simulink model "testes_com_trajetorias"  (R2016a)
settings: Solver=ode14x  StartTime=0.0  StopTime=30  FixedStep=0.001  RelTol=1e-3
InitFcn:
  | clear all;
  | Kpx = 10;
  | Kix = 25;
  | Kpy = 10;
  | Kiy = 25;
  | Kvphi = 3;
  | Kpphi = 2.25;
  | 
  | Kem = 0.0059;
  | Kti = 0.0059;
  | Vd = 5.4;
  | R = 1.71;
  | r = 0.072;
  | eta = 0.83;
  | N = 19;
  | 
  | Jw = 8.1e-4;
  | 
  | mi = 0.25;
  | b = .1;
  | 
  | Ts = 0.01;
  | 
  | 
  | alpha1 = 0;
  | alpha2 = 120*pi/180;
  | alpha3 = 240*pi/180;
  | g = 9.8;
  | vs = 6e-10;
  | M = 1.83;
  | l1 = 0.09;
  | l2 = 0.09;
  | l3 = 0.09;
  | r1 = 0.072;
  | r2 = 0.072;
  | r3 = 0.072;
  | kt = 0.0059;
  | kem = 0.0059;
  | N = 19;
  | L = 0.00011;
  | R = 1.71;
  | Jm1 = 3.88e-7;
  | Jm2 = 3.88e-7;
  | Jm3 = 3.88e-7;
  | J1 = 8.1e-4;
  | J2 = 8.1e-4;
  | J3 = 8.1e-4;
  | J = 2.125;
  | eta = 0.83;
  | freq = 1000; % varia entre 2.5kHz e 5Mhz
  | mic = 0.25;
  | mis = 0.25;
  | sigma0 = 100;
  | sigma1 = 0.1;
  | sigma2 = 0.1;
  | 
  | mi = 0.25;
  | b = .1;
  | 
  | kctr = kt*5.4*eta*N/(R*r1)
libraries: simulink x2
settings Model: Creator=Pichau  LastModifiedBy=Pichau

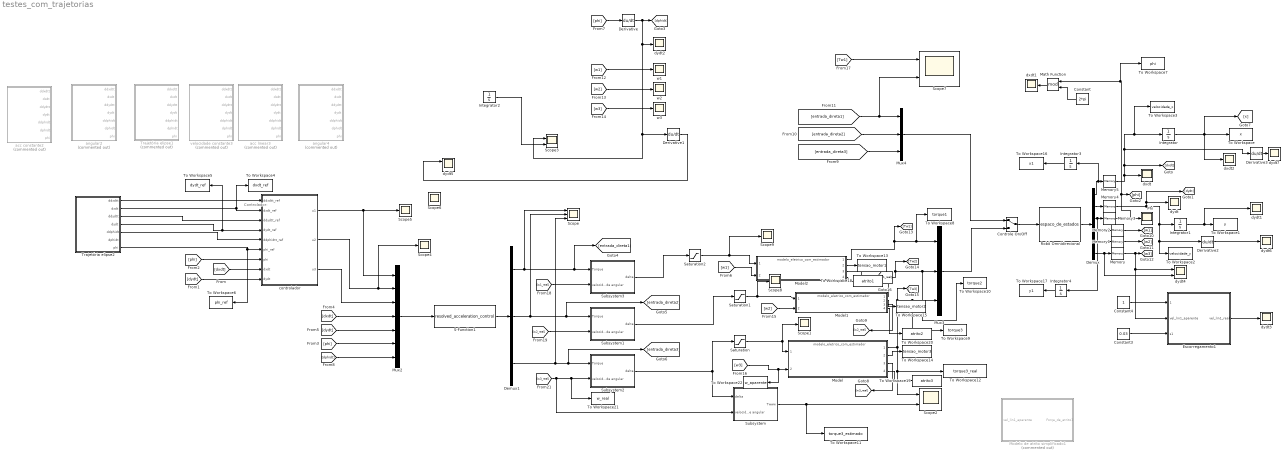
== system testes_com_trajetorias ==
  note: Controlador:
  Constant : Constant  Value=2*pi
  Constant3 : Constant  Value=0.03
  Constant4 : Constant
  Controle On/Off : ManualSwitch
  Demux : Demux  Outputs=6
  Demux1 : Demux  Outputs=3
  Derivative{,1..3} (4 alike) : Derivative
  Escorregamento1 : Subsystem
  Integrator : Integrator  InitialCondition=0.3
  Integrator{1..4} (4 alike) : Integrator
  Math Function : Math  Operator=mod  SaturateOnIntegerOverflow=on
  Memory{,1..2,4..5} (5 alike) : Memory
  Memory3 : Memory  X0=pi/2
  Model : ModelReference  ModelNameDialog=modelo_eletrico_com_estimador  SimulationMode=Normal  ModelReferenceVersion=1.40
  Model1 : ModelReference  ModelNameDialog=modelo_eletrico_com_estimador  SimulationMode=Normal  ModelReferenceVersion=1.40
  Model2 : ModelReference  ModelNameDialog=modelo_eletrico_com_estimador  SimulationMode=Normal  ModelReferenceVersion=1.40
  Modelo de atrito simplificado1 : Subsystem  Commented=on
  Mux2 : Mux  Inputs=7
  Mux3 : Mux  Inputs=3
  Mux4 : Mux  Inputs=3
  Phi : Scope
  Robô Omnidirecional : S-Function  FunctionName=espaco_de_estados  Parameters=r,m,Jw,J,L  SFunctionDeploymentMode=off  EnableBusSupport=off  mask{r=0.072, m=1.71, Jw=8.1e-4, J=2.125, L=0.09}
      mask prompts: r "r (m)"; m "m (Kg)"; Jw "Jw (Kg*m^2)"; J "J (Kg*m^2)"; L "L (m)"
      mask Display: image(imread('Robot_omnidirectional_drive.png'));
  S-Function1 : S-Function  FunctionName=resolved_acceleration_control  Parameters=r,L,m,J,Jw  SFunctionDeploymentMode=off  EnableBusSupport=off  mask{r=0.072, L=0.09, m=1.71, J=2.125, Jw=8.1e-4}
  Saturation : Saturate  UpperLimit=1  LowerLimit=-1
  Saturation1 : Saturate  UpperLimit=1  LowerLimit=-1
  Saturation2 : Saturate  UpperLimit=1  LowerLimit=-1
  Scope : Scope  NumInputPorts=3
  Scope{1,4..6,8..9} (6 alike) : Scope
  Scope2 : Scope  NumInputPorts=2
  Scope3 : Scope  NumInputPorts=2
  Scope7 : Scope  NumInputPorts=2
  Subsystem : Subsystem
  Subsystem1 : Subsystem
  Subsystem2 : Subsystem
  Subsystem3 : Subsystem
  To Workspace : ToWorkspace  VariableName=x  SaveFormat=Timeseries  SampleTime=-1
  To Workspace1 : ToWorkspace  VariableName=y  SaveFormat=Timeseries  SampleTime=-1
  To Workspace10 : ToWorkspace  VariableName=torque2  SaveFormat=Timeseries  SampleTime=-1
  To Workspace11 : ToWorkspace  VariableName=torque3_estimado  SaveFormat=Timeseries  SampleTime=-1
  To Workspace12 : ToWorkspace  VariableName=torque3_real  SaveFormat=Timeseries  SampleTime=-1
  To Workspace13 : ToWorkspace  VariableName=tensao_motor1  SaveFormat=Timeseries  SampleTime=-1
  To Workspace14 : ToWorkspace  VariableName=tensao_motor3  SaveFormat=Timeseries  SampleTime=-1
  To Workspace15 : ToWorkspace  VariableName=tensao_motor2  SaveFormat=Timeseries  SampleTime=-1
  To Workspace16 : ToWorkspace  VariableName=x1  SaveFormat=Timeseries  SampleTime=-1
  To Workspace17 : ToWorkspace  VariableName=y1  SaveFormat=Timeseries  SampleTime=-1
  To Workspace18 : ToWorkspace  VariableName=atrito1  SaveFormat=Timeseries  SampleTime=-1
  To Workspace19 : ToWorkspace  VariableName=atrito3  SaveFormat=Timeseries  SampleTime=-1
  To Workspace2 : ToWorkspace  VariableName=velocidade_y  SaveFormat=Timeseries  SampleTime=-1
  To Workspace20 : ToWorkspace  VariableName=atrito2  SaveFormat=Timeseries  SampleTime=-1
  To Workspace21 : ToWorkspace  VariableName=w_real  SaveFormat=Timeseries  SampleTime=-1
  To Workspace22 : ToWorkspace  VariableName=w_aparente  SaveFormat=Timeseries  SampleTime=-1
  To Workspace3 : ToWorkspace  VariableName=velocidade_x  SaveFormat=Timeseries  SampleTime=-1
  To Workspace4 : ToWorkspace  VariableName=dxdt_ref  SaveFormat=Timeseries  SampleTime=-1
  To Workspace5 : ToWorkspace  VariableName=dydt_ref  SaveFormat=Timeseries  SampleTime=-1
  To Workspace6 : ToWorkspace  VariableName=phi_ref  SaveFormat=Timeseries  SampleTime=-1
  To Workspace7 : ToWorkspace  VariableName=phi  SaveFormat=Timeseries  SampleTime=-1
  To Workspace8 : ToWorkspace  VariableName=torque1  SaveFormat=Timeseries  SampleTime=-1
  To Workspace9 : ToWorkspace  VariableName=torque3  SaveFormat=Timeseries  SampleTime=-1
  Trajetória elipse1 : Subsystem  Commented=on
  Trajetória elipse2 : Subsystem
  acc constante2 : Subsystem  Commented=on
  acc linear3 : Subsystem  Commented=on
  angular2 : Subsystem  Commented=on
  angular4 : Subsystem  Commented=on
  controlador : Subsystem
  dxdt : Scope
  dxdt1 : Scope
  dxdt2 : Scope
  dydt{,1..3,6..7} (6 alike) : Scope
  dydt4 : Scope  NumInputPorts=2
  dydt5 : Scope  NumInputPorts=2
  velocidade constante3 : Subsystem  Commented=on
  w1 : Scope
  w2 : Scope
  w3 : Scope
  wires:
  Robô Omnidirecional/1 -> Demux/1
  Integrator1/1 -> dydt1/1, To Workspace1/1
  Integrator/1 -> dxdt2/1, [x], To Workspace/1
  Trajetória elipse2/2(dxdt) -> controlador/2(dxdt_ref), To Workspace4/1
  Trajetória elipse2/1(ddxdtt) -> controlador/1(ddxdtt_ref)
  Trajetória elipse2/4(dydt) -> To Workspace5/1, controlador/4(dydt_ref)
  Trajetória elipse2/3(ddydtt) -> controlador/3(ddydtt_ref)
  Trajetória elipse2/7(phi) -> To Workspace6/1, controlador/6(phi_ref)
  Trajetória elipse2/5(ddphidt) -> controlador/5(ddphidtt_ref)
  [dxdt] -> controlador/8(dxdt)
  [dydt] -> controlador/9(dydt)
  [phi] -> controlador/7(phi)
  Mux2/1 -> S-Function1/1
  Derivative/1 -> Scope3/1, Derivative1/1, dydt2/1, [dphidt]
  S-Function1/1 -> Demux1/1
  Mux3/1 -> Controle On/Off/2
  Controle On/Off/1 -> Robô Omnidirecional/1
  [w3] -> w3/1
  [w2] -> w2/1
  [w1] -> w1/1
  Demux/1 -> Integrator3/1, Memory5/1
  Demux/2 -> Memory4/1
  [phi] -> Derivative/1
  [dxdt] -> Mux2/4
  [dydt] -> Mux2/5
  [phi] -> Mux2/6
  [dphidt] -> Mux2/7
  Demux/4 -> Memory2/1
  Demux/5 -> Memory1/1
  Demux/6 -> dydt4/2, Memory/1
  Model/1 -> [Tw3], Mux3/3, To Workspace9/1, Scope2/1, To Workspace12/1
  Model1/1 -> [Tw2], To Workspace10/1, Mux3/2
  Model2/1 -> [Tw1], To Workspace8/1, Mux3/1
  Mux4/1 -> Controle On/Off/1
  Demux1/1 -> Scope/1, Subsystem3/1(Torque), [entrada_direta1]
  Subsystem1/1(delta) -> Saturation1/1
  Subsystem3/1(delta) -> Saturation2/1
  [w1_real] -> Subsystem3/2(velocidade angular)
  [w2_real] -> Subsystem1/2(velocidade angular)
  [w3_real] -> Subsystem/2(velocidade angular), To Workspace21/1, Subsystem2/2(velocidade angular)
  Constant3/1 -> Escorregamento1/3(s1)
  Constant4/1 -> Escorregamento1/1(1)
  Escorregamento1/1("vel_lin1_real ") -> dydt3/1
  Memory/1 -> Escorregamento1/2("vel_lin1_aparente "), dydt4/1, [w3]
  Memory1/1 -> [w2]
  Memory2/1 -> [w1]
  Memory4/1 -> To Workspace2/1, Derivative2/1, Integrator1/1, [dydt], dydt/1
  Memory5/1 -> [dxdt], Derivative3/1, To Workspace3/1, Integrator/1, dxdt/1
  Subsystem2/1(delta) -> Subsystem/1(delta), Saturation/1
  Subsystem/1(Twww) -> To Workspace11/1, Scope2/2
  Demux1/2 -> Scope/2, Subsystem1/1(Torque), [entrada_direta2]
  Demux1/3 -> Scope/3, [entrada_direta3], Subsystem2/1(Torque)
  Math Function/1 -> dxdt1/1
  Constant/1 -> Math Function/2
  Memory3/1 -> Phi/1, [phi], To Workspace7/1, Math Function/1
  Saturation/1 -> Scope1/1, Model/1
  Saturation1/1 -> Scope8/1, Model1/1
  [entrada_direta3] -> Mux4/3
  [entrada_direta2] -> Mux4/2
  Integrator2/1 -> Scope3/2
  Derivative1/1 -> dydt5/1
  Derivative2/1 -> dydt6/1
  Derivative3/1 -> dydt7/1
  controlador/2(u2) -> Scope4/1, Mux2/2
  controlador/1(u1) -> Mux2/1, Scope5/1
  controlador/3(u3) -> Mux2/3
  [w1] -> Model2/2
  [w2] -> Model1/2
  [w3] -> To Workspace22/1, Model/2
  [Tw1] -> Scope7/1
  [entrada_direta1] -> Scope7/2, Mux4/1
  Saturation2/1 -> Scope9/1, Model2/1
  Model2/2 -> To Workspace13/1
  Model1/2 -> To Workspace15/1
  Model/2 -> To Workspace14/1
  Integrator3/1 -> To Workspace16/1
  Demux/3 -> Integrator4/1, Memory3/1
  Integrator4/1 -> To Workspace17/1
  Model/3 -> [w3_real]
  Model1/3 -> [w2_real]
  Model2/3 -> [w1_real]
  Model2/4 -> To Workspace18/1
  Model1/4 -> To Workspace20/1
  Model/4 -> To Workspace19/1

== system testes_com_trajetorias/Escorregamento1 ==
  1 : Inport
  "vel_lin1_aparente " : Inport  Port=2
  s1 : Inport  Port=3
  Fcn : Fcn  Expr=1/u[1]
  Product : Product  RndMeth=Zero
  Sum3 : Sum  Inputs=+|+
  Sum4 : Sum  Inputs=|+-
  Switch : Switch
  "vel_lin1_real " : Outport
  wires:
  s1/1 -> Switch/2, Sum3/1, Sum4/2
  1/1 -> Sum3/2, Sum4/1
  Sum4/1 -> Fcn/1
  Fcn/1 -> Switch/1
  Sum3/1 -> Switch/3
  Switch/1 -> Product/2
  "vel_lin1_aparente "/1 -> Product/1
  Product/1 -> "vel_lin1_real "/1

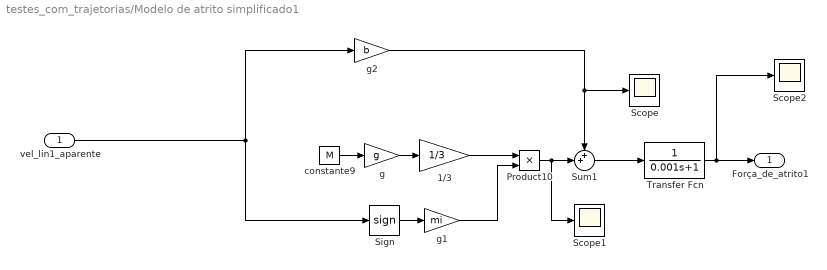
== system testes_com_trajetorias/Modelo de atrito simplificado1 ==
  vel_lin1_aparente : Inport
  1/3 : Gain  Gain=1/3
  Product10 : Product  RndMeth=Zero
  Scope : Scope
  Scope1 : Scope
  Scope2 : Scope
  Sign : Signum
  Sum1 : Sum  Inputs=++|
  Transfer Fcn : TransferFcn  Denominator=[0.001 1]
  constante9 : Constant  Value=M
  g : Gain  Gain=g
  g1 : Gain  Gain=mi
  g2 : Gain  Gain=b
  Força_de_atrito1 : Outport
  wires:
  Transfer Fcn/1 -> Força_de_atrito1/1, Scope2/1
  g2/1 -> Scope/1, Sum1/1
  Sum1/1 -> Transfer Fcn/1
  Sign/1 -> g1/1
  vel_lin1_aparente/1 -> Sign/1, g2/1
  Product10/1 -> Sum1/2, Scope1/1
  g1/1 -> Product10/2
  1/3/1 -> Product10/1
  g/1 -> 1/3/1
  constante9/1 -> g/1

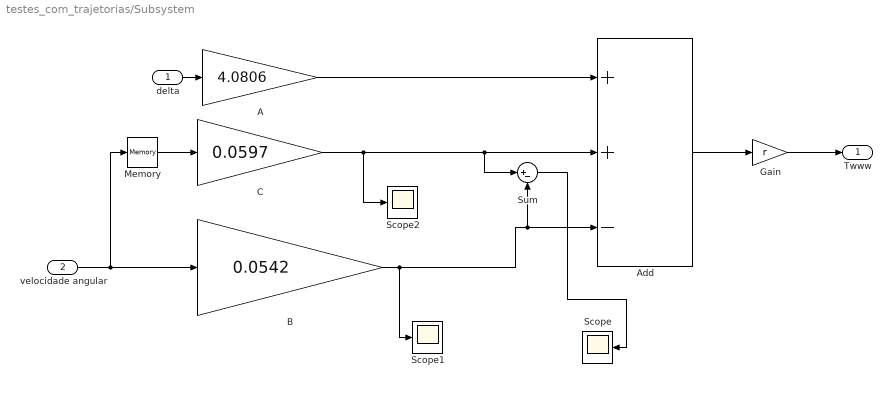
== system testes_com_trajetorias/Subsystem ==
  delta : Inport
  velocidade angular : Inport  Port=2
  A : Gain  Gain=4.0806
  Add : Sum  Inputs=++-
  B : Gain  Gain=0.0542
  C : Gain  Gain=0.0597
  Gain : Gain  Gain=r
  Memory : Memory
  Scope : Scope
  Scope1 : Scope
  Scope2 : Scope
  Sum : Sum  Inputs=|+-
  Twww : Outport
  wires:
  Add/1 -> Gain/1
  delta/1 -> A/1
  velocidade angular/1 -> Memory/1, B/1
  A/1 -> Add/1
  Memory/1 -> C/1
  Gain/1 -> Twww/1
  C/1 -> Scope2/1, Sum/1, Add/2
  Sum/1 -> Scope/1
  B/1 -> Scope1/1, Add/3, Sum/2

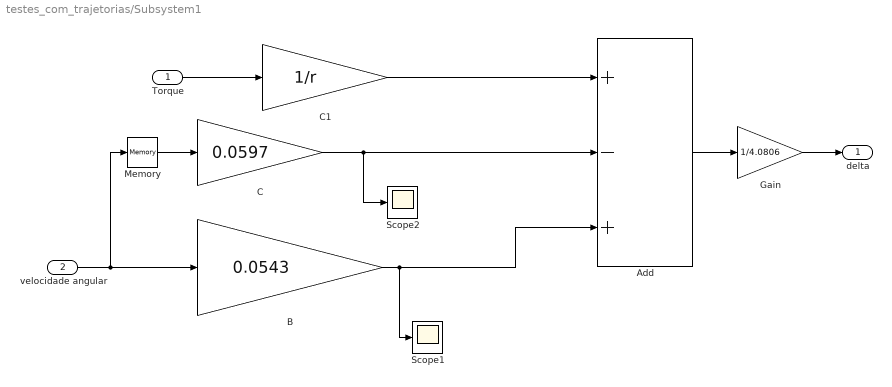
== system testes_com_trajetorias/Subsystem1 ==
  Torque : Inport
  velocidade angular : Inport  Port=2
  Add : Sum  Inputs=+-+
  B : Gain  Gain=0.0543
  C : Gain  Gain=0.0597
  C1 : Gain  Gain=1/r
  Gain : Gain  Gain=1/4.0806
  Memory : Memory
  Scope1 : Scope
  Scope2 : Scope
  delta : Outport
  wires:
  C1/1 -> Add/1
  Add/1 -> Gain/1
  velocidade angular/1 -> Memory/1, B/1
  Torque/1 -> C1/1
  Memory/1 -> C/1
  Gain/1 -> delta/1
  C/1 -> Scope2/1, Add/2
  B/1 -> Scope1/1, Add/3

== system testes_com_trajetorias/Subsystem2 ==
  Torque : Inport
  velocidade angular : Inport  Port=2
  Add : Sum  Inputs=+-+
  B : Gain  Gain=0.0543
  C : Gain  Gain=0.0597
  C1 : Gain  Gain=1/r
  Gain : Gain  Gain=1/4.0806
  Memory : Memory
  Scope1 : Scope
  Scope2 : Scope
  delta : Outport
  wires:
  B/1 -> Add/3, Scope1/1
  C/1 -> Add/2, Scope2/1
  Gain/1 -> delta/1
  Memory/1 -> C/1
  Torque/1 -> C1/1
  velocidade angular/1 -> B/1, Memory/1
  Add/1 -> Gain/1
  C1/1 -> Add/1

== system testes_com_trajetorias/Subsystem3 ==
  Torque : Inport
  velocidade angular : Inport  Port=2
  Add : Sum  Inputs=+-+
  B : Gain  Gain=0.0543
  C : Gain  Gain=0.0597
  C1 : Gain  Gain=1/r
  Gain : Gain  Gain=1/4.0806
  Memory : Memory
  Scope1 : Scope
  Scope2 : Scope
  delta : Outport
  wires:
  B/1 -> Add/3, Scope1/1
  C/1 -> Add/2, Scope2/1
  Gain/1 -> delta/1
  Memory/1 -> C/1
  Torque/1 -> C1/1
  velocidade angular/1 -> B/1, Memory/1
  Add/1 -> Gain/1
  C1/1 -> Add/1

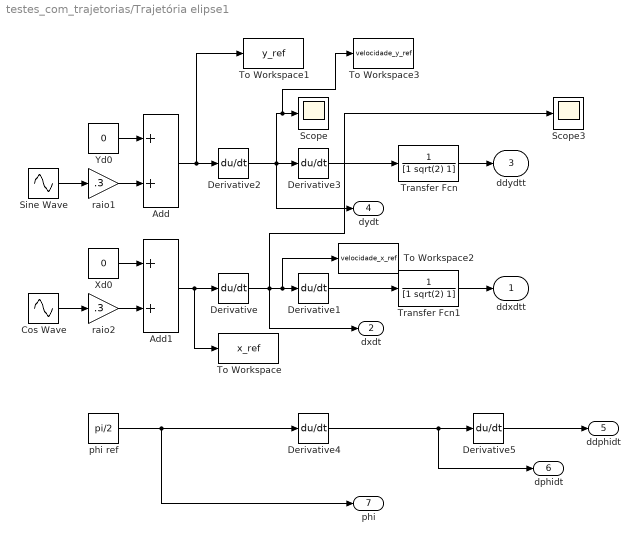
== system testes_com_trajetorias/Trajetória elipse1 ==
  Add : Sum
  Add1 : Sum
  Cos Wave : Sin  Frequency=0.3  Phase=pi/2  SampleTime=0
  Derivative{,1..5} (6 alike) : Derivative
  Scope : Scope
  Scope3 : Scope
  Sine Wave : Sin  Frequency=0.3  SampleTime=0
  To Workspace : ToWorkspace  VariableName=x_ref  SaveFormat=Timeseries  SampleTime=-1
  To Workspace1 : ToWorkspace  VariableName=y_ref  SaveFormat=Timeseries  SampleTime=-1
  To Workspace2 : ToWorkspace  VariableName=velocidade_x_ref  SaveFormat=Timeseries  SampleTime=-1
  To Workspace3 : ToWorkspace  VariableName=velocidade_y_ref  SaveFormat=Timeseries  SampleTime=-1
  Transfer Fcn : TransferFcn  Denominator=[1 sqrt(2) 1]
  Transfer Fcn1 : TransferFcn  Denominator=[1 sqrt(2) 1]
  Xd0 : Constant  Value=0
  Yd0 : Constant  Value=0
  phi ref : Constant  Value=pi/2
  raio1 : Gain  Gain=.3
  raio2 : Gain  Gain=.3
  ddxdtt : Outport
  dxdt : Outport  Port=2
  ddydtt : Outport  Port=3
  dydt : Outport  Port=4
  ddphidt : Outport  Port=5
  dphidt : Outport  Port=6
  phi : Outport  Port=7
  wires:
  Derivative4/1 -> dphidt/1, Derivative5/1
  phi ref/1 -> phi/1, Derivative4/1
  Yd0/1 -> Add/1
  Xd0/1 -> Add1/1
  Cos Wave/1 -> raio2/1
  raio2/1 -> Add1/2
  Add1/1 -> Derivative/1, To Workspace/1
  Add/1 -> Derivative2/1, To Workspace1/1
  raio1/1 -> Add/2
  Sine Wave/1 -> raio1/1
  Derivative/1 -> dxdt/1, Derivative1/1, To Workspace2/1, Scope3/1
  Derivative2/1 -> dydt/1, Scope/1, To Workspace3/1, Derivative3/1
  Derivative3/1 -> Transfer Fcn/1
  Derivative1/1 -> Transfer Fcn1/1
  Derivative5/1 -> ddphidt/1
  Transfer Fcn/1 -> ddydtt/1
  Transfer Fcn1/1 -> ddxdtt/1

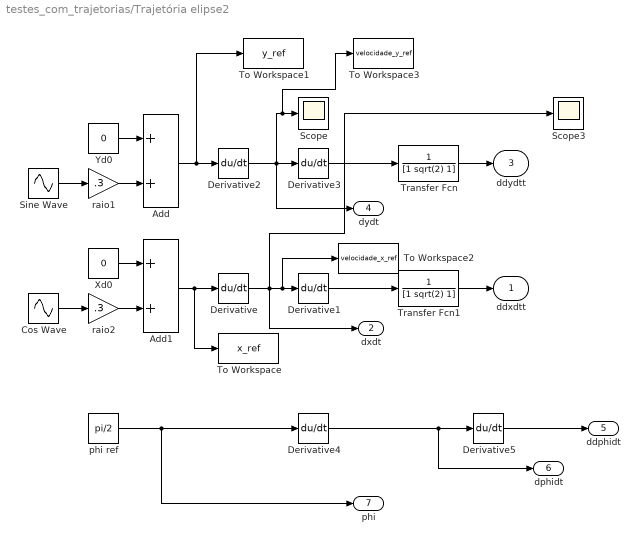
== system testes_com_trajetorias/Trajetória elipse2 ==
  Add : Sum
  Add1 : Sum
  Cos Wave : Sin  Frequency=0.3  Phase=pi/2  SampleTime=0
  Derivative{,1..5} (6 alike) : Derivative
  Scope : Scope
  Scope3 : Scope
  Sine Wave : Sin  Frequency=0.3  SampleTime=0
  To Workspace : ToWorkspace  VariableName=x_ref  SaveFormat=Timeseries  SampleTime=-1
  To Workspace1 : ToWorkspace  VariableName=y_ref  SaveFormat=Timeseries  SampleTime=-1
  To Workspace2 : ToWorkspace  VariableName=velocidade_x_ref  SaveFormat=Timeseries  SampleTime=-1
  To Workspace3 : ToWorkspace  VariableName=velocidade_y_ref  SaveFormat=Timeseries  SampleTime=-1
  Transfer Fcn : TransferFcn  Denominator=[1 sqrt(2) 1]
  Transfer Fcn1 : TransferFcn  Denominator=[1 sqrt(2) 1]
  Xd0 : Constant  Value=0
  Yd0 : Constant  Value=0
  phi ref : Constant  Value=pi/2
  raio1 : Gain  Gain=.3
  raio2 : Gain  Gain=.3
  ddxdtt : Outport
  dxdt : Outport  Port=2
  ddydtt : Outport  Port=3
  dydt : Outport  Port=4
  ddphidt : Outport  Port=5
  dphidt : Outport  Port=6
  phi : Outport  Port=7
  wires:
  Transfer Fcn1/1 -> ddxdtt/1
  Transfer Fcn/1 -> ddydtt/1
  Derivative5/1 -> ddphidt/1
  Derivative1/1 -> Transfer Fcn1/1
  Derivative3/1 -> Transfer Fcn/1
  Derivative2/1 -> Derivative3/1, To Workspace3/1, Scope/1, dydt/1
  Derivative/1 -> Scope3/1, To Workspace2/1, Derivative1/1, dxdt/1
  Sine Wave/1 -> raio1/1
  raio1/1 -> Add/2
  Add/1 -> To Workspace1/1, Derivative2/1
  Add1/1 -> To Workspace/1, Derivative/1
  raio2/1 -> Add1/2
  Cos Wave/1 -> raio2/1
  Xd0/1 -> Add1/1
  Yd0/1 -> Add/1
  phi ref/1 -> Derivative4/1, phi/1
  Derivative4/1 -> Derivative5/1, dphidt/1

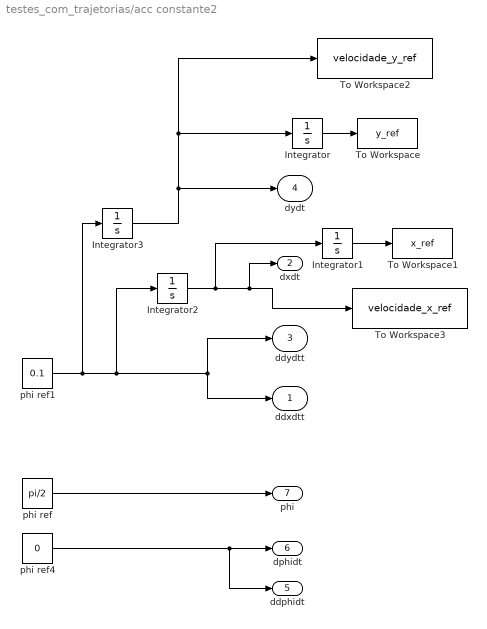
== system testes_com_trajetorias/acc constante2 ==
  Integrator{,1..3} (4 alike) : Integrator
  To Workspace : ToWorkspace  VariableName=y_ref  SaveFormat=Timeseries  SampleTime=-1
  To Workspace1 : ToWorkspace  VariableName=x_ref  SaveFormat=Timeseries  SampleTime=-1
  To Workspace2 : ToWorkspace  VariableName=velocidade_y_ref  SaveFormat=Timeseries  SampleTime=-1
  To Workspace3 : ToWorkspace  VariableName=velocidade_x_ref  SaveFormat=Timeseries  SampleTime=-1
  phi ref : Constant  Value=pi/2
  phi ref1 : Constant  Value=0.1
  phi ref4 : Constant  Value=0
  ddxdtt : Outport
  dxdt : Outport  Port=2
  ddydtt : Outport  Port=3
  dydt : Outport  Port=4
  ddphidt : Outport  Port=5
  dphidt : Outport  Port=6
  phi : Outport  Port=7
  wires:
  Integrator2/1 -> To Workspace3/1, dxdt/1, Integrator1/1
  Integrator1/1 -> To Workspace1/1
  Integrator/1 -> To Workspace/1
  Integrator3/1 -> dydt/1, To Workspace2/1, Integrator/1
  phi ref1/1 -> ddxdtt/1, ddydtt/1, Integrator2/1, Integrator3/1
  phi ref/1 -> phi/1
  phi ref4/1 -> ddphidt/1, dphidt/1

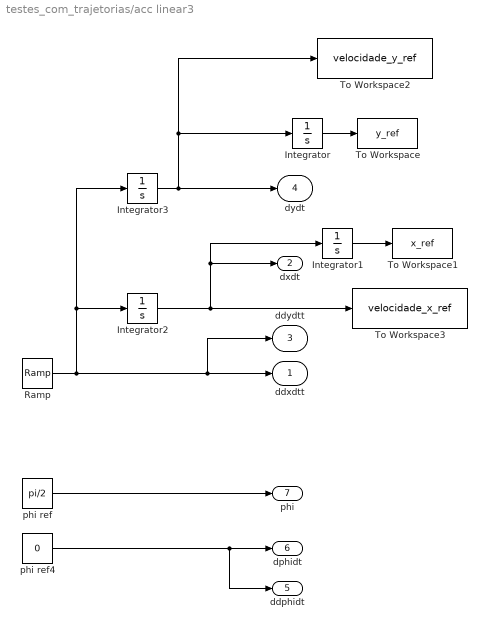
== system testes_com_trajetorias/acc linear3 ==
  Integrator{,1..3} (4 alike) : Integrator
  Ramp : simulink/Sources/Ramp  slope=0.01  start=0  X0=0
  To Workspace : ToWorkspace  VariableName=y_ref  SaveFormat=Timeseries  SampleTime=-1
  To Workspace1 : ToWorkspace  VariableName=x_ref  SaveFormat=Timeseries  SampleTime=-1
  To Workspace2 : ToWorkspace  VariableName=velocidade_y_ref  SaveFormat=Timeseries  SampleTime=-1
  To Workspace3 : ToWorkspace  VariableName=velocidade_x_ref  SaveFormat=Timeseries  SampleTime=-1
  phi ref : Constant  Value=pi/2
  phi ref4 : Constant  Value=0
  ddxdtt : Outport
  dxdt : Outport  Port=2
  ddydtt : Outport  Port=3
  dydt : Outport  Port=4
  ddphidt : Outport  Port=5
  dphidt : Outport  Port=6
  phi : Outport  Port=7
  wires:
  Integrator3/1 -> dydt/1, To Workspace2/1, Integrator/1
  Integrator1/1 -> To Workspace1/1
  Integrator/1 -> To Workspace/1
  Ramp/1 -> Integrator2/1, Integrator3/1, ddxdtt/1, ddydtt/1
  Integrator2/1 -> To Workspace3/1, dxdt/1, Integrator1/1
  phi ref/1 -> phi/1
  phi ref4/1 -> ddphidt/1, dphidt/1

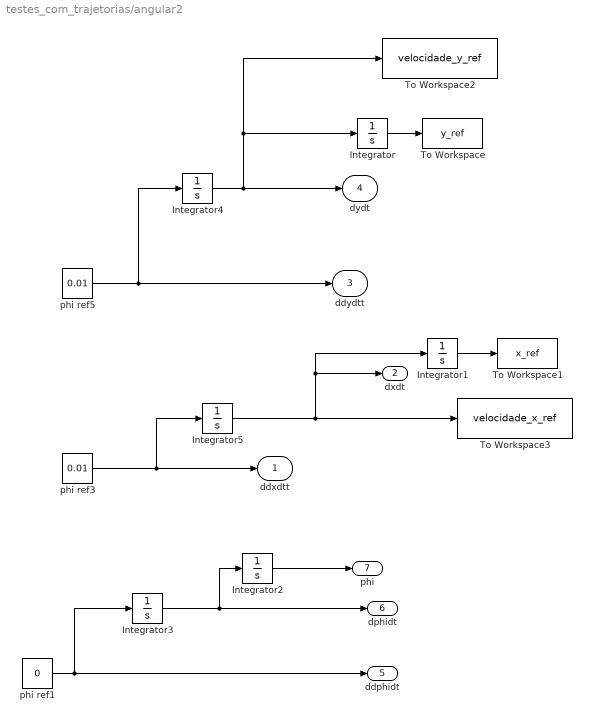
== system testes_com_trajetorias/angular2 ==
  Integrator : Integrator
  Integrator1 : Integrator
  Integrator2 : Integrator  InitialCondition=pi/4
  Integrator3 : Integrator  InitialCondition=pi/18
  Integrator4 : Integrator  InitialCondition=0.1
  Integrator5 : Integrator  InitialCondition=0.1
  To Workspace : ToWorkspace  VariableName=y_ref  SaveFormat=Timeseries  SampleTime=-1
  To Workspace1 : ToWorkspace  VariableName=x_ref  SaveFormat=Timeseries  SampleTime=-1
  To Workspace2 : ToWorkspace  VariableName=velocidade_y_ref  SaveFormat=Timeseries  SampleTime=-1
  To Workspace3 : ToWorkspace  VariableName=velocidade_x_ref  SaveFormat=Timeseries  SampleTime=-1
  phi ref1 : Constant  Value=0
  phi ref3 : Constant  Value=0.01
  phi ref5 : Constant  Value=0.01
  ddxdtt : Outport
  dxdt : Outport  Port=2
  ddydtt : Outport  Port=3
  dydt : Outport  Port=4
  ddphidt : Outport  Port=5
  dphidt : Outport  Port=6
  phi : Outport  Port=7
  wires:
  phi ref3/1 -> ddxdtt/1, Integrator5/1
  phi ref1/1 -> ddphidt/1, Integrator3/1
  Integrator3/1 -> Integrator2/1, dphidt/1
  Integrator1/1 -> To Workspace1/1
  Integrator/1 -> To Workspace/1
  Integrator4/1 -> dydt/1, To Workspace2/1, Integrator/1
  Integrator5/1 -> To Workspace3/1, dxdt/1, Integrator1/1
  phi ref5/1 -> Integrator4/1, ddydtt/1
  Integrator2/1 -> phi/1

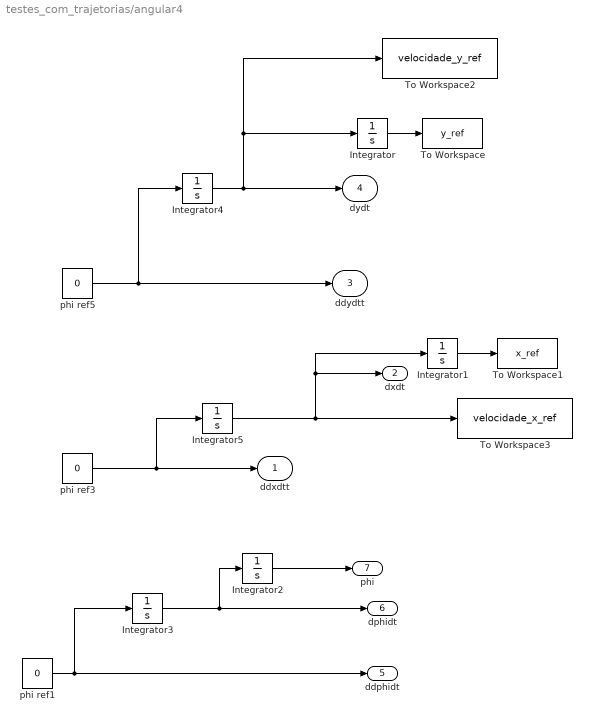
== system testes_com_trajetorias/angular4 ==
  Integrator : Integrator
  Integrator1 : Integrator
  Integrator2 : Integrator
  Integrator3 : Integrator  InitialCondition=0.1521
  Integrator4 : Integrator  InitialCondition=0.1
  Integrator5 : Integrator  InitialCondition=0.1
  To Workspace : ToWorkspace  VariableName=y_ref  SaveFormat=Timeseries  SampleTime=-1
  To Workspace1 : ToWorkspace  VariableName=x_ref  SaveFormat=Timeseries  SampleTime=-1
  To Workspace2 : ToWorkspace  VariableName=velocidade_y_ref  SaveFormat=Timeseries  SampleTime=-1
  To Workspace3 : ToWorkspace  VariableName=velocidade_x_ref  SaveFormat=Timeseries  SampleTime=-1
  phi ref1 : Constant  Value=0
  phi ref3 : Constant  Value=0
  phi ref5 : Constant  Value=0
  ddxdtt : Outport
  dxdt : Outport  Port=2
  ddydtt : Outport  Port=3
  dydt : Outport  Port=4
  ddphidt : Outport  Port=5
  dphidt : Outport  Port=6
  phi : Outport  Port=7
  wires:
  phi ref3/1 -> ddxdtt/1, Integrator5/1
  phi ref1/1 -> ddphidt/1, Integrator3/1
  Integrator3/1 -> Integrator2/1, dphidt/1
  Integrator1/1 -> To Workspace1/1
  Integrator/1 -> To Workspace/1
  Integrator4/1 -> dydt/1, To Workspace2/1, Integrator/1
  Integrator5/1 -> To Workspace3/1, dxdt/1, Integrator1/1
  phi ref5/1 -> Integrator4/1, ddydtt/1
  Integrator2/1 -> phi/1

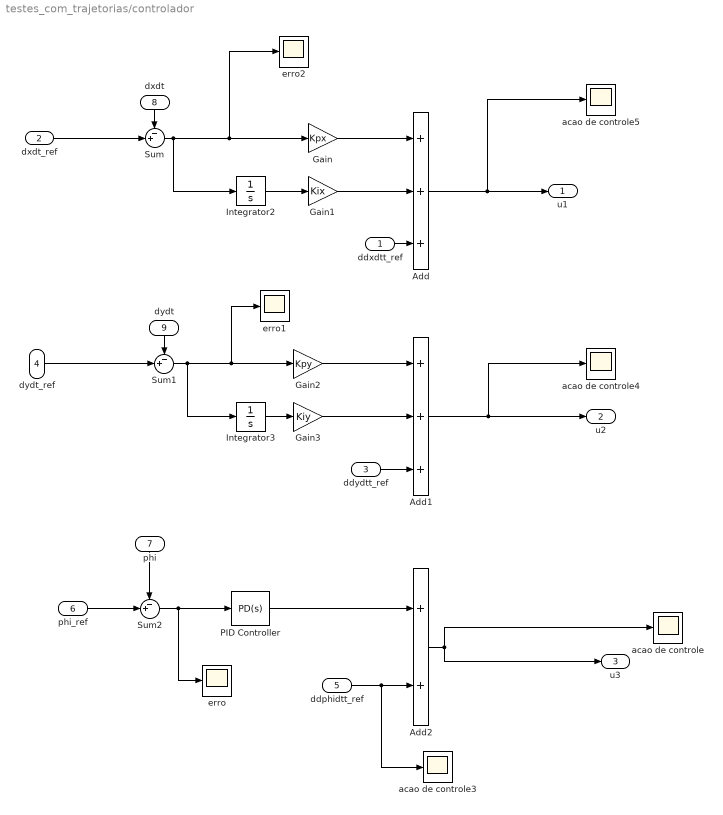
== system testes_com_trajetorias/controlador ==
  ddxdtt_ref : Inport
  dxdt_ref : Inport  Port=2
  ddydtt_ref : Inport  Port=3
  dydt_ref : Inport  Port=4
  ddphidtt_ref : Inport  Port=5
  phi_ref : Inport  Port=6
  phi : Inport  Port=7
  dxdt : Inport  Port=8
  dydt : Inport  Port=9
  Add : Sum  Inputs=+++
  Add1 : Sum  Inputs=+++
  Add2 : Sum
  Gain : Gain  Gain=Kpx
  Gain1 : Gain  Gain=Kix
  Gain2 : Gain  Gain=Kpy
  Gain3 : Gain  Gain=Kiy
  Integrator2 : Integrator
  Integrator3 : Integrator
  PID Controller : simulink/Continuous/PID Controller  Controller=PD  TimeDomain=Continuous-time  SampleTime=-1  IntegratorMethod=Forward Euler  FilterMethod=Forward Euler  Form=Parallel  UseFilter=on  ControllerParametersSource=internal  P=2.25  I=0  D=3  N=100  InitialConditionSource=internal  InitialConditionForIntegrator=0  InitialConditionForFilter=0  ExternalReset=none  LimitOutput=off  UpperSaturationLimit=inf  LowerSaturationLimit=-inf  LinearizeAsGain=on  AntiWindupMode=none  Kb=1  TrackingMode=off  Kt=1  PParamMin=[]  PParamMax=[]  IParamMin=[]  IParamMax=[]  DParamMin=[]  DParamMax=[]  NParamMin=[]  NParamMax=[]  KbParamMin=[]  KbParamMax=[]  KtParamMin=[]  KtParamMax=[]  POutMin=[]  POutMax=[]  IOutMin=[]  IOutMax=[]  DOutMin=[]  DOutMax=[]  NOutMin=[]  NOutMax=[]  KbOutMin=[]  KbOutMax=[]  KtOutMin=[]  KtOutMax=[]  IntegratorOutMin=[]  IntegratorOutMax=[]  FilterOutMin=[]  FilterOutMax=[]  SumOutMin=[]  SumOutMax=[]  SumI1OutMin=[]  SumI1OutMax=[]  SumI2OutMin=[]  SumI2OutMax=[]  SumI3OutMin=[]  SumI3OutMax=[]  SumDOutMin=[]  SumDOutMax=[]  SaturationOutMin=[]  SaturationOutMax=[]  IntegratorContinuousStateAttributes=''  IntegratorStateMustResolveToSignalObject=off  IntegratorRTWStateStorageClass=Auto  FilterContinuousStateAttributes=''  FilterStateMustResolveToSignalObject=off  FilterRTWStateStorageClass=Auto  DifferentiatorICPrevScaledInput=0  DifferentiatorOutMin=[]  DifferentiatorOutMax=[]
  Sum : Sum  Inputs=-+|
  Sum1 : Sum  Inputs=-+|
  Sum2 : Sum  Inputs=-+|
  acao de controle{,3..5} (4 alike) : Scope
  erro : Scope
  erro1 : Scope
  erro2 : Scope
  u1 : Outport
  u2 : Outport  Port=2
  u3 : Outport  Port=3
  wires:
  Sum2/1 -> erro/1, PID Controller/1
  Sum1/1 -> erro1/1, Gain2/1, Integrator3/1
  Gain1/1 -> Add/2
  Integrator2/1 -> Gain1/1
  dydt_ref/1 -> Sum1/2
  Gain2/1 -> Add1/1
  Integrator3/1 -> Gain3/1
  Sum/1 -> erro2/1, Gain/1, Integrator2/1
  Gain3/1 -> Add1/2
  ddphidtt_ref/1 -> acao de controle3/1, Add2/2
  ddydtt_ref/1 -> Add1/3
  ddxdtt_ref/1 -> Add/3
  phi/1 -> Sum2/1
  dxdt_ref/1 -> Sum/2
  dxdt/1 -> Sum/1
  phi_ref/1 -> Sum2/2
  Gain/1 -> Add/1
  dydt/1 -> Sum1/1
  Add1/1 -> acao de controle4/1, u2/1
  Add/1 -> acao de controle5/1, u1/1
  Add2/1 -> u3/1, acao de controle/1
  PID Controller/1 -> Add2/1

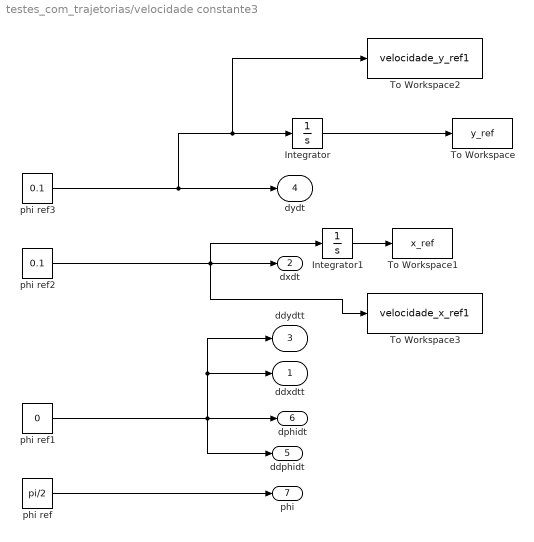
== system testes_com_trajetorias/velocidade constante3 ==
  Integrator : Integrator
  Integrator1 : Integrator
  To Workspace : ToWorkspace  VariableName=y_ref  SaveFormat=Timeseries  SampleTime=-1
  To Workspace1 : ToWorkspace  VariableName=x_ref  SaveFormat=Timeseries  SampleTime=-1
  To Workspace2 : ToWorkspace  VariableName=velocidade_y_ref1  SaveFormat=Timeseries  SampleTime=-1
  To Workspace3 : ToWorkspace  VariableName=velocidade_x_ref1  SaveFormat=Timeseries  SampleTime=-1
  phi ref : Constant  Value=pi/2
  phi ref1 : Constant  Value=0
  phi ref2 : Constant  Value=0.1
  phi ref3 : Constant  Value=0.1
  ddxdtt : Outport
  dxdt : Outport  Port=2
  ddydtt : Outport  Port=3
  dydt : Outport  Port=4
  ddphidt : Outport  Port=5
  dphidt : Outport  Port=6
  phi : Outport  Port=7
  wires:
  Integrator1/1 -> To Workspace1/1
  Integrator/1 -> To Workspace/1
  phi ref3/1 -> dydt/1, To Workspace2/1, Integrator/1
  phi ref2/1 -> To Workspace3/1, dxdt/1, Integrator1/1
  phi ref1/1 -> dphidt/1, ddphidt/1, ddxdtt/1, ddydtt/1
  phi ref/1 -> phi/1
